simulink model "stm32f0_ccp_sensor"  (Simulink 7.3)
settings: Solver=ode3  SolverMode=SingleTasking  StartTime=0.0  StopTime=10.0  RelTol=1e-3
PreLoadFcn:
  | waijung.modelPreload; % Required for working with Waijung Blockset. Do not remove.
undefined symbols (not defined in the file): ARM, LQFP48, MDK, STM32F072CB
libraries: simulink x216, waijung_soft_i2c_lib x28, waijung_addon_module x12, stm32f0_flash_lib x10, stm32f0_can_lib x3, stm32f0_reset_lib x1, waijung_crc_lib x1, stm32f0_boot_lib x1, stm32f0_device_config_lib x1
(part 2 of 6)

== system stm32f0_ccp_sensor/CCP Handler/CRO CONNECT Parser ==
  Data(8) : Inport  OutDataType=fixdt(1, 16)  OutScaling=2^0
  CONNECT Handler : Subsystem  TreatAsAtomicUnit=on
  Demux : Demux  Outputs=8
  Mux : Mux  Inputs=6
  Terminator : Terminator
  Connected : Outport  OutDataType=fixdt(1, 16)  OutScaling=2^0
  CMD : Outport  Port=2  OutDataType=fixdt(1, 16)  OutScaling=2^0
  Data(6) : Outport  Port=3  OutDataType=fixdt(1, 16)  OutScaling=2^0
  CTR : Outport  Port=4  OutDataType=fixdt(1, 16)  OutScaling=2^0
  wires:
  Data(8)/1 -> Demux/1
  Demux/1 -> CMD/1, CONNECT Handler/1(CMD)
  Demux/3 -> CONNECT Handler/2(Station Addr LSB), Mux/1
  Demux/4 -> CONNECT Handler/3(Station Addr MSB), Mux/2
  CONNECT Handler/1(Connected) -> Connected/1
  CONNECT Handler/2(Station Address) -> Terminator/1
  Demux/8 -> Mux/6
  Demux/7 -> Mux/5
  Demux/6 -> Mux/4
  Demux/5 -> Mux/3
  Mux/1 -> Data(6)/1
  Demux/2 -> CTR/1

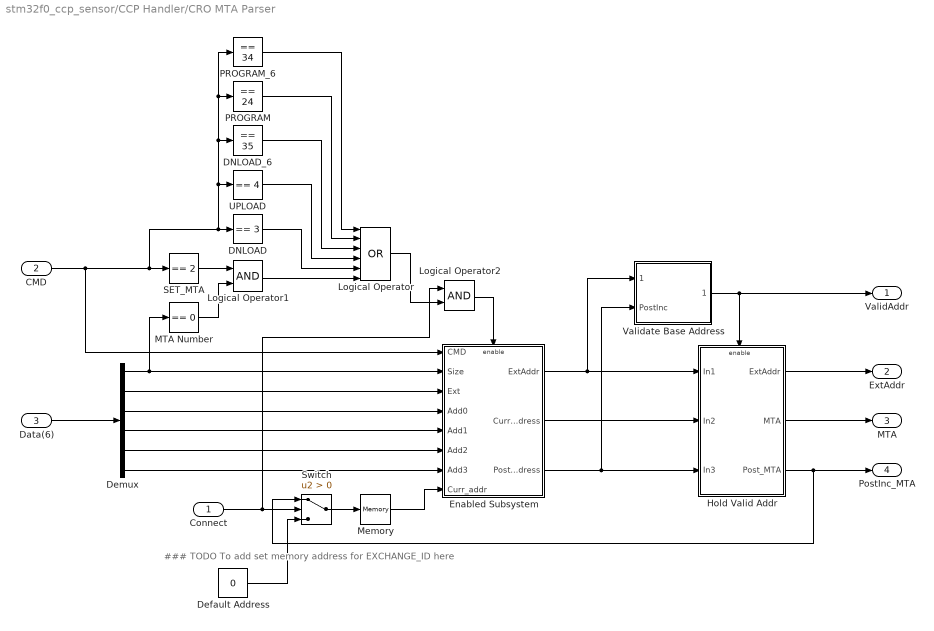
== system stm32f0_ccp_sensor/CCP Handler/CRO MTA Parser ==
  note: ### TODO
      | To add set memory address for EXCHANGE_ID here
  Connect : Inport  OutDataType=fixdt(1, 16)  OutScaling=2^0
  CMD : Inport  Port=2  OutDataType=fixdt(1, 16)  OutScaling=2^0
  Data(6) : Inport  Port=3  OutDataType=fixdt(1, 16)  OutScaling=2^0
  DNLOAD : simulink/Logic and Bit Operations/Compare To Constant  SystemSampleTime=-1  relop===  const=3  LogicOutDataTypeMode=uint8  ZeroCross=off
  DNLOAD_6 : simulink/Logic and Bit Operations/Compare To Constant  SystemSampleTime=-1  relop===  const=35  LogicOutDataTypeMode=uint8  ZeroCross=off
  Default Address : Constant  Value=0  OutDataTypeMode=uint32  OutDataType=fixdt(1, 16)  OutScaling=2^0  OutDataTypeStr=uint32
  Demux : Demux  Outputs=6
  Enabled Subsystem : Subsystem  TreatAsAtomicUnit=on
  Hold Valid Addr : Subsystem
  Logical Operator : Logic  Operator=OR  Inputs=6  AllPortsSameDT=off  OutDataTypeMode=boolean  LogicDataType=fixdt(0, 8)  OutDataTypeStr=boolean
  Logical Operator1 : Logic  AllPortsSameDT=off  OutDataTypeMode=boolean  LogicDataType=fixdt(0, 8)  OutDataTypeStr=boolean
  Logical Operator2 : Logic  AllPortsSameDT=off  OutDataTypeMode=boolean  LogicDataType=fixdt(0, 8)  OutDataTypeStr=boolean
  MTA Number : simulink/Logic and Bit Operations/Compare To Constant  SystemSampleTime=-1  relop===  const=0  LogicOutDataTypeMode=uint8  ZeroCross=off
  Memory : Memory  InheritSampleTime=on  LinearizeMemory=on
  PROGRAM : simulink/Logic and Bit Operations/Compare To Constant  SystemSampleTime=-1  relop===  const=24  LogicOutDataTypeMode=uint8  ZeroCross=off
  PROGRAM_6 : simulink/Logic and Bit Operations/Compare To Constant  SystemSampleTime=-1  relop===  const=34  LogicOutDataTypeMode=uint8  ZeroCross=off
  SET_MTA : simulink/Logic and Bit Operations/Compare To Constant  SystemSampleTime=-1  relop===  const=2  LogicOutDataTypeMode=uint8  ZeroCross=off
  Switch : Switch  Criteria=u2 > Threshold  OutDataType=fixdt(1, 16)  OutScaling=2^0
  UPLOAD : simulink/Logic and Bit Operations/Compare To Constant  SystemSampleTime=-1  relop===  const=4  LogicOutDataTypeMode=uint8  ZeroCross=off
  Validate Base Address : Subsystem
  ValidAddr : Outport  OutDataType=fixdt(1, 16)  OutScaling=2^0
  ExtAddr : Outport  Port=2  OutDataType=fixdt(1, 16)  OutScaling=2^0
  MTA : Outport  Port=3  OutDataType=fixdt(1, 16)  OutScaling=2^0
  PostInc_MTA : Outport  Port=4  OutDataType=fixdt(1, 16)  OutScaling=2^0
  wires:
  Data(6)/1 -> Demux/1
  CMD/1 -> SET_MTA/1, DNLOAD/1, UPLOAD/1, DNLOAD_6/1, PROGRAM/1, PROGRAM_6/1, Enabled Subsystem/1(CMD)
  Demux/1 -> MTA Number/1, Enabled Subsystem/2(Size)
  MTA Number/1 -> Logical Operator1/2
  SET_MTA/1 -> Logical Operator1/1
  Demux/3 -> Enabled Subsystem/4(Add0)
  Demux/4 -> Enabled Subsystem/5(Add1)
  Demux/5 -> Enabled Subsystem/6(Add2)
  Demux/6 -> Enabled Subsystem/7(Add3)
  Demux/2 -> Enabled Subsystem/3(Ext)
  Enabled Subsystem/2(Curr_Address) -> Hold Valid Addr/2(In2)
  Logical Operator1/1 -> Logical Operator/6
  PROGRAM_6/1 -> Logical Operator/1
  PROGRAM/1 -> Logical Operator/2
  DNLOAD_6/1 -> Logical Operator/3
  UPLOAD/1 -> Logical Operator/4
  DNLOAD/1 -> Logical Operator/5
  Enabled Subsystem/3(Post_Address) -> Hold Valid Addr/3(In3), Validate Base Address/2(PostInc)
  Memory/1 -> Enabled Subsystem/8(Curr_addr)
  Switch/1 -> Memory/1
  Connect/1 -> Switch/2, Logical Operator2/1
  Default Address/1 -> Switch/3
  Logical Operator2/1 -> Enabled Subsystem/Enable
  Logical Operator/1 -> Logical Operator2/2
  Enabled Subsystem/1(ExtAddr) -> Hold Valid Addr/1(In1), Validate Base Address/1(ExtAddr)
  Hold Valid Addr/1(ExtAddr) -> ExtAddr/1
  Hold Valid Addr/2(MTA) -> MTA/1
  Hold Valid Addr/3(Post_MTA) -> PostInc_MTA/1, Switch/1
  Validate Base Address/1(ValidAddr) -> Hold Valid Addr/Enable, ValidAddr/1

== system stm32f0_ccp_sensor/CCP Handler/CRO UNLOCK Parser ==
  Connect : Inport  OutDataType=fixdt(1, 16)  OutScaling=2^0
  CMD : Inport  Port=2  OutDataType=fixdt(1, 16)  OutScaling=2^0
  Data(6) : Inport  Port=3  OutDataType=fixdt(1, 16)  OutScaling=2^0
  Constant : Constant  Value=[0 0 0]  OutDataTypeMode=uint8  OutDataType=fixdt(1, 16)  OutScaling=2^0  OutDataTypeStr=uint8
  Demux : Demux  Outputs=3
  Enabled Subsystem : Subsystem  TreatAsAtomicUnit=on
  Memory : Memory
  Switch : Switch  Criteria=u2 > Threshold  OutDataType=fixdt(1, 16)  OutScaling=2^0
  CAL Unlocked : Outport  OutDataType=fixdt(1, 16)  OutScaling=2^0
  PGM Unlocked : Outport  Port=2  OutDataType=fixdt(1, 16)  OutScaling=2^0
  DAQ Unlocked : Outport  Port=3  OutDataType=fixdt(1, 16)  OutScaling=2^0
  wires:
  Connect/1 -> Switch/2, Enabled Subsystem/Enable
  Constant/1 -> Switch/3
  Switch/1 -> Demux/1, Memory/1
  Demux/1 -> CAL Unlocked/1
  Demux/2 -> PGM Unlocked/1
  Demux/3 -> DAQ Unlocked/1
  Memory/1 -> Enabled Subsystem/3(Last status)
  Data(6)/1 -> Enabled Subsystem/2(Data(6))
  CMD/1 -> Enabled Subsystem/1(CMD)
  Enabled Subsystem/1(Out1) -> Switch/1

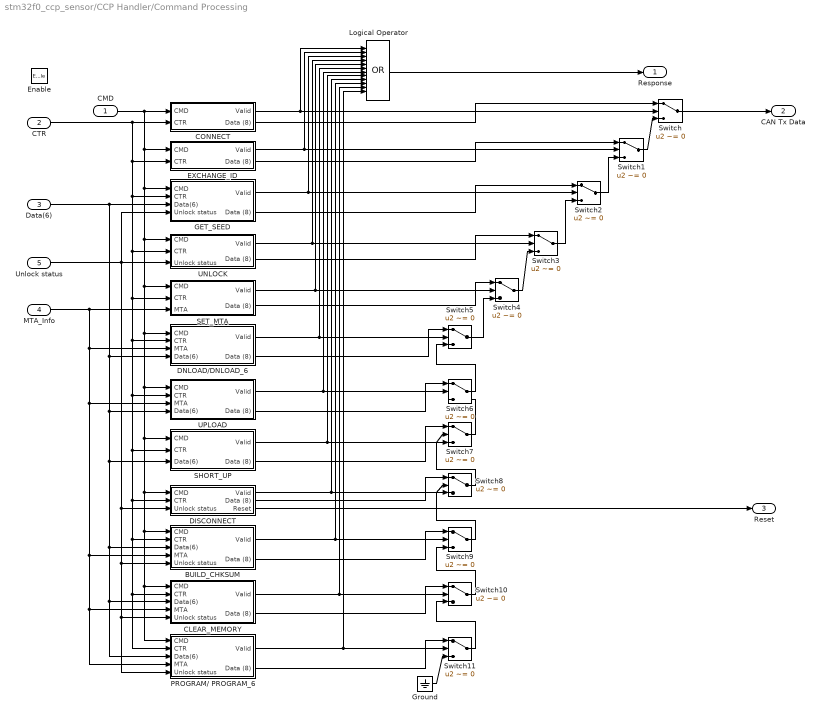
== system stm32f0_ccp_sensor/CCP Handler/Command Processing ==
  CMD : Inport  OutDataType=fixdt(1, 16)  OutScaling=2^0
  CTR : Inport  Port=2  OutDataType=fixdt(1, 16)  OutScaling=2^0
  Data(6) : Inport  Port=3  OutDataType=fixdt(1, 16)  OutScaling=2^0
  MTA_Info : Inport  Port=4  OutDataType=fixdt(1, 16)  OutScaling=2^0
  Unlock status : Inport  Port=5  OutDataType=fixdt(1, 16)  OutScaling=2^0
  Enable : EnablePort
  BUILD_CHKSUM : Subsystem
  CLEAR_MEMORY : Subsystem
  CONNECT : Subsystem
  DISCONNECT : Subsystem
  DNLOAD/DNLOAD_6 : Subsystem
  EXCHANGE_ID : Subsystem
  GET_SEED : Subsystem
  Ground : Ground
  Logical Operator : Logic  Operator=OR  Inputs=12  AllPortsSameDT=off  OutDataTypeMode=boolean  LogicDataType=fixdt(0, 8)  OutDataTypeStr=boolean
  PROGRAM/ PROGRAM_6 : Subsystem
  SET_MTA : Subsystem
  SHORT_UP : Subsystem
  Switch{,1..11} (12 alike) : Switch  Criteria=u2 ~= 0  OutDataType=fixdt(1, 16)  OutScaling=2^0
  UNLOCK : Subsystem
  UPLOAD : Subsystem
  Response : Outport  OutDataType=fixdt(1, 16)  OutScaling=2^0
  CAN Tx Data : Outport  Port=2  OutDataType=fixdt(1, 16)  OutScaling=2^0  InitialOutput=[0 0 0 0 0 0 0 0]
  Reset : Outport  Port=3  OutDataType=fixdt(1, 16)  OutScaling=2^0  InitialOutput=0
  wires:
  CMD/1 -> CONNECT/1(CMD), EXCHANGE_ID/1(CMD), GET_SEED/1(CMD), UNLOCK/1(CMD), SET_MTA/1(CMD), UPLOAD/1(CMD), SHORT_UP/1(CMD), DISCONNECT/1(CMD), BUILD_CHKSUM/1(CMD), CLEAR_MEMORY/1(CMD), PROGRAM/ PROGRAM_6/1(CMD), DNLOAD/DNLOAD_6/1(CMD)
  Switch/1 -> CAN Tx Data/1
  CTR/1 -> CONNECT/2(CTR), EXCHANGE_ID/2(CTR), GET_SEED/2(CTR), UNLOCK/2(CTR), SET_MTA/2(CTR), DNLOAD/DNLOAD_6/2(CTR), UPLOAD/2(CTR), SHORT_UP/2(CTR), DISCONNECT/2(CTR), BUILD_CHKSUM/2(CTR), CLEAR_MEMORY/2(CTR), PROGRAM/ PROGRAM_6/2(CTR)
  CONNECT/1(Valid) -> Logical Operator/1, Switch/2
  EXCHANGE_ID/1(Valid) -> Logical Operator/2, Switch1/2
  Data(6)/1 -> GET_SEED/3(Data(6)), DNLOAD/DNLOAD_6/4(Data(6)), UPLOAD/4(Data(6)), SHORT_UP/3(Data(6)), BUILD_CHKSUM/3(Data(6)), CLEAR_MEMORY/3(Data(6)), PROGRAM/ PROGRAM_6/3(Data(6))
  GET_SEED/1(Valid) -> Logical Operator/3, Switch2/2
  Switch2/1 -> Switch1/3
  GET_SEED/2(Data (8)) -> Switch2/1
  EXCHANGE_ID/2(Data (8)) -> Switch1/1
  CONNECT/2(Data (8)) -> Switch/1
  Switch1/1 -> Switch/3
  Logical Operator/1 -> Response/1
  Unlock status/1 -> GET_SEED/4(Unlock status), UNLOCK/3(Unlock status), BUILD_CHKSUM/5(Unlock status), CLEAR_MEMORY/5(Unlock status), PROGRAM/ PROGRAM_6/5(Unlock status), DISCONNECT/3(Unlock status)
  UNLOCK/1(Valid) -> Logical Operator/4, Switch3/2
  Switch3/1 -> Switch2/3
  UNLOCK/2(Data (8)) -> Switch3/1
  SET_MTA/1(Valid) -> Logical Operator/5, Switch4/2
  Switch4/1 -> Switch3/3
  SET_MTA/2(Data (8)) -> Switch4/1
  MTA_Info/1 -> SET_MTA/3(MTA), DNLOAD/DNLOAD_6/3(MTA), UPLOAD/3(MTA), BUILD_CHKSUM/4(MTA), CLEAR_MEMORY/4(MTA), PROGRAM/ PROGRAM_6/4(MTA)
  DNLOAD/DNLOAD_6/1(Valid) -> Logical Operator/6, Switch5/2
  Switch5/1 -> Switch4/3
  DNLOAD/DNLOAD_6/2(Data (8)) -> Switch5/1
  UPLOAD/1(Valid) -> Logical Operator/7, Switch6/2
  Switch6/1 -> Switch5/3
  UPLOAD/2(Data (8)) -> Switch6/1
  SHORT_UP/1(Valid) -> Logical Operator/8, Switch7/2
  Switch7/1 -> Switch6/3
  SHORT_UP/2(Data (8)) -> Switch7/1
  DISCONNECT/1(Valid) -> Logical Operator/9, Switch8/2
  Switch8/1 -> Switch7/3
  DISCONNECT/2(Data (8)) -> Switch8/1
  BUILD_CHKSUM/1(Valid) -> Logical Operator/10, Switch9/2
  BUILD_CHKSUM/2(Data (8)) -> Switch9/1
  Switch9/1 -> Switch8/3
  CLEAR_MEMORY/1(Valid) -> Logical Operator/11, Switch10/2
  Switch10/1 -> Switch9/3
  CLEAR_MEMORY/2(Data (8)) -> Switch10/1
  PROGRAM/ PROGRAM_6/1(Valid) -> Logical Operator/12, Switch11/2
  PROGRAM/ PROGRAM_6/2(Data (8)) -> Switch11/1
  Switch11/1 -> Switch10/3
  Ground/1 -> Switch11/3
  DISCONNECT/3(Reset) -> Reset/1

== system stm32f0_ccp_sensor/HIH6131/Read ==
  In1 : Inport
  Enable : EnablePort
  Compare To Zero : simulink/Logic and Bit Operations/Compare To Zero  SystemSampleTime=-1  relop===  LogicOutDataTypeMode=boolean  ZeroCross=off
  Constant1 : Constant  Value=40  OutDataTypeMode=single  OutDataType=fixdt(1, 16)  OutScaling=2^0  OutDataTypeStr=single
  Data Type Conversion3 : DataTypeConversion  OutDataTypeMode=single  OutDataType=fixdt(1, 16)  OutScaling=2^0  OutDataTypeStr=single
  Data Type Conversion4 : DataTypeConversion  OutDataTypeMode=single  OutDataType=fixdt(1, 16)  OutScaling=2^0  OutDataTypeStr=single
  Gain : Gain  Gain=100/16382  ParameterDataType=fixdt(1, 16)  ParameterScaling=2^0  OutDataType=fixdt(1, 16)  OutScaling=2^0
  Gain1 : Gain  Gain=165/16382  ParameterDataType=fixdt(1, 16)  ParameterScaling=2^0  OutDataType=fixdt(1, 16)  OutScaling=2^0
  Mux : Mux
  Soft I2C Master Read/Write : waijung_soft_i2c_lib/Soft I2C Master Read//Write  conf=ReadWrite  targetname=stm32f0  module=1  transfer=Blocking  clk=100  timeout=25  sdapins={'A4','A6'}  sclpins='A5'  writecount=0  readcount=4  waittime=0  forcestop=off  portpinstr=0  sampletime=inf  blockid=HIH6131ReadSoftI2CMasterReadWrite  inputporttype=[3]  inputportwidth=[]  inputportlabel={'SlvAddr'}  outputporttype="[3 3 3 3 3    ]"  outputportwidth=[1 1 1 1 1]  outputportlabel={'Status' 'Rd0 (uint8)' 'Rd1 (uint8)' 'Rd2 (uint8)' 'Rd3 (uint8)'}  compat=0  optionstring="[\"1\",\"0\",\"4\",\"0\",\"off\",\"1\"]"
  Subsystem : Subsystem
  Subtract : Sum  Inputs=+-  OutDataType=fixdt(1, 16)  OutScaling=2^-10
  Terminator : Terminator
  Humid : Outport  OutDataType=fixdt(1, 16)  OutScaling=2^0
  Temp : Outport  Port=2  OutDataType=fixdt(1, 16)  OutScaling=2^0
  wires:
  Soft I2C Master Read/Write/2 -> Mux/1
  Soft I2C Master Read/Write/3 -> Mux/2
  Soft I2C Master Read/Write/4 -> Mux/3
  Soft I2C Master Read/Write/5 -> Mux/4
  Mux/1 -> Subsystem/1(In1)
  Compare To Zero/1 -> Subsystem/Enable
  Soft I2C Master Read/Write/1 -> Compare To Zero/1
  Subsystem/2(Humidity) -> Data Type Conversion3/1
  Subsystem/3(Temperature) -> Data Type Conversion4/1
  Gain1/1 -> Subtract/1
  Constant1/1 -> Subtract/2
  Subsystem/1(Status) -> Terminator/1
  Subtract/1 -> Temp/1
  Data Type Conversion3/1 -> Gain/1
  Data Type Conversion4/1 -> Gain1/1
  Gain/1 -> Humid/1
  In1/1 -> Soft I2C Master Read/Write/1

== system stm32f0_ccp_sensor/HIH6131/Request ==
  In1 : Inport
  Enable : EnablePort
  Soft I2C Master Read/Write : waijung_soft_i2c_lib/Soft I2C Master Read//Write  conf=ReadWrite  targetname=stm32f0  module=1  transfer=Blocking  clk=100  timeout=25  sdapins={'A4','A6'}  sclpins='A5'  writecount=0  readcount=0  waittime=0  forcestop=off  portpinstr=0  sampletime=inf  blockid=HIH6131RequestSoftI2CMasterReadWrite  inputporttype=[3]  inputportwidth=[]  inputportlabel={'SlvAddr'}  outputporttype=[3]  outputportwidth=[1]  outputportlabel={'Status'}  compat=0  optionstring="[\"1\",\"0\",\"0\",\"0\",\"off\",\"1\"]"
  Terminator : Terminator
  wires:
  In1/1 -> Soft I2C Master Read/Write/1
  Soft I2C Master Read/Write/1 -> Terminator/1

== system stm32f0_ccp_sensor/MAX44009/Enabled Subsystem ==
  note: # E
  note: #M
  Configuration : Inport  OutDataType=fixdt(1, 16)  OutScaling=2^0
  MSB : Inport  Port=2  OutDataType=fixdt(1, 16)  OutScaling=2^0
  LSB : Inport  Port=3  OutDataType=fixdt(1, 16)  OutScaling=2^0
  Enable : EnablePort
  Bitwise Operator : simulink/Logic and Bit Operations/Bitwise Operator  logicop=OR  UseBitMask=off  NumInputPorts=2  BitMask=bin2dec('11011001')  BitMaskRealWorld=Stored Integer
  Bitwise Operator1 : simulink/Logic and Bit Operations/Bitwise Operator  logicop=AND  UseBitMask=on  BitMask=hex2dec('F')  BitMaskRealWorld=Stored Integer
  CDR_ : simulink/Logic and Bit Operations/Bitwise Operator  logicop=AND  UseBitMask=on  BitMask=8  BitMaskRealWorld=Stored Integer
  Compare To Zero : simulink/Logic and Bit Operations/Compare To Zero  SystemSampleTime=-1  relop=~=  LogicOutDataTypeMode=uint8  ZeroCross=off
  Constant1 : Constant  Value=0.045  OutDataType=fixdt(1, 16)  OutScaling=2^0
  Constant2 : Constant  Value=2  OutDataTypeMode=single  OutDataType=fixdt(1, 16)  OutScaling=2^0  OutDataTypeStr=single
  Data Type Conversion{,1..3} (4 alike) : DataTypeConversion  OutDataTypeMode=single  OutDataType=fixdt(1, 16)  OutScaling=2^0  OutDataTypeStr=single
  Math Function : Math  Operator=pow  OutDataType=fixdt(1, 16)  OutScaling=2^0  SaturateOnIntegerOverflow=on
  Product : Product  Inputs=3  OutDataType=fixdt(1, 16)  OutScaling=2^0  RndMeth=Zero  OutDataTypeStr=Inherit: Same as first input
  Shift Arithmetic : simulink/Logic and Bit Operations/Shift Arithmetic  SystemSampleTime=-1  nBitShiftRight=4  nBinPtShiftRight=0
  Shift Arithmetic1 : simulink/Logic and Bit Operations/Shift Arithmetic  SystemSampleTime=-1  nBitShiftRight=-4  nBinPtShiftRight=0
  Lux : Outport  OutDataType=fixdt(1, 16)  OutScaling=2^0
  CDR : Outport  Port=2  OutDataType=fixdt(1, 16)  OutScaling=2^0
  wires:
  Compare To Zero/1 -> CDR/1
  CDR_/1 -> Compare To Zero/1
  Data Type Conversion2/1 -> Product/1
  Data Type Conversion/1 -> Product/2
  Bitwise Operator1/1 -> Data Type Conversion3/1
  Constant1/1 -> Data Type Conversion2/1
  Math Function/1 -> Data Type Conversion/1
  MSB/1 -> Shift Arithmetic/1, Shift Arithmetic1/1
  Shift Arithmetic/1 -> Bitwise Operator1/1
  Shift Arithmetic1/1 -> Bitwise Operator/1
  LSB/1 -> Bitwise Operator/2
  Bitwise Operator/1 -> Data Type Conversion1/1
  Data Type Conversion1/1 -> Product/3
  Configuration/1 -> CDR_/1
  Product/1 -> Lux/1
  Constant2/1 -> Math Function/1
  Data Type Conversion3/1 -> Math Function/2

== system stm32f0_ccp_sensor/MPL3115A2/Convert ==
  In1 : Inport
  In2 : Inport  Port=2
  In3 : Inport  Port=3
  Enable : EnablePort
  Add : Sum  OutDataType=fixdt(1, 16)  OutScaling=2^-10
  Bitwise Operator : simulink/Logic and Bit Operations/Bitwise Operator  logicop=OR  UseBitMask=off  NumInputPorts=3  BitMask=bin2dec('11011001')  BitMaskRealWorld=Stored Integer
  Bitwise Operator1 : simulink/Logic and Bit Operations/Bitwise Operator  logicop=AND  UseBitMask=on  BitMask=3  BitMaskRealWorld=Stored Integer
  Data Type Conversion{,1..2,4} (4 alike) : DataTypeConversion  OutDataTypeMode=uint32  OutDataType=fixdt(1, 16)  OutScaling=2^0  OutDataTypeStr=uint32
  Data Type Conversion3 : DataTypeConversion  OutDataTypeMode=single  OutDataType=fixdt(1, 16)  OutScaling=2^0  OutDataTypeStr=single
  Data Type Conversion6 : DataTypeConversion  OutDataTypeMode=single  OutDataType=fixdt(1, 16)  OutScaling=2^0  OutDataTypeStr=single
  Gain : Gain  Gain=0.25  ParameterDataType=fixdt(1, 16)  ParameterScaling=2^0  OutDataTypeMode=single  OutDataType=fixdt(1, 16)  OutScaling=2^0  OutDataTypeStr=single
  Shift Arithmetic : simulink/Logic and Bit Operations/Shift Arithmetic  SystemSampleTime=-1  nBitShiftRight=-10  nBinPtShiftRight=0
  Shift Arithmetic1 : simulink/Logic and Bit Operations/Shift Arithmetic  SystemSampleTime=-1  nBitShiftRight=4  nBinPtShiftRight=0
  Shift Arithmetic2 : simulink/Logic and Bit Operations/Shift Arithmetic  SystemSampleTime=-1  nBitShiftRight=-2  nBinPtShiftRight=0
  Shift Arithmetic3 : simulink/Logic and Bit Operations/Shift Arithmetic  SystemSampleTime=-1  nBitShiftRight=6  nBinPtShiftRight=0
  Pa : Outport  OutDataType=fixdt(1, 16)  OutScaling=2^0
  wires:
  Shift Arithmetic3/1 -> Bitwise Operator/3
  Data Type Conversion4/1 -> Shift Arithmetic3/1
  Shift Arithmetic2/1 -> Bitwise Operator/2
  In3/1 -> Data Type Conversion4/1, Shift Arithmetic1/1
  In2/1 -> Data Type Conversion1/1
  Add/1 -> Pa/1
  In1/1 -> Data Type Conversion/1
  Data Type Conversion6/1 -> Add/2
  Gain/1 -> Data Type Conversion6/1
  Data Type Conversion3/1 -> Add/1
  Bitwise Operator1/1 -> Gain/1
  Shift Arithmetic1/1 -> Bitwise Operator1/1
  Data Type Conversion2/1 -> Data Type Conversion3/1
  Bitwise Operator/1 -> Data Type Conversion2/1
  Data Type Conversion1/1 -> Shift Arithmetic2/1
  Shift Arithmetic/1 -> Bitwise Operator/1
  Data Type Conversion/1 -> Shift Arithmetic/1

== system stm32f0_ccp_sensor/MPL3115A2/MPL3115A2_Initialize ==
  SlvAddr : Inport  OutDataType=fixdt(1, 16)  OutScaling=2^0
  CNTRL_REG1 : Constant  Value=hex2dec('26')  OutDataTypeMode=uint8  OutDataType=fixdt(1, 16)  OutScaling=2^0  OutDataTypeStr=uint8
  Compare To Constant : simulink/Logic and Bit Operations/Compare To Constant  SystemSampleTime=-1  relop===  const=7  LogicOutDataTypeMode=boolean  ZeroCross=off
  Compare To Constant1 : simulink/Logic and Bit Operations/Compare To Constant  SystemSampleTime=-1  relop===  const=hex2dec('39')  LogicOutDataTypeMode=boolean  ZeroCross=off
  Compare To Zero : simulink/Logic and Bit Operations/Compare To Zero  SystemSampleTime=-1  relop===  LogicOutDataTypeMode=boolean  ZeroCross=off
  Compare To Zero1 : simulink/Logic and Bit Operations/Compare To Zero  SystemSampleTime=-1  relop===  LogicOutDataTypeMode=boolean  ZeroCross=off
  Logical Operator1 : Logic  Inputs=4  AllPortsSameDT=off  OutDataTypeMode=boolean  LogicDataType=fixdt(0, 8)  OutDataTypeStr=boolean
  Logical Operator2 : Logic  Inputs=3  AllPortsSameDT=off  OutDataTypeMode=boolean  LogicDataType=fixdt(0, 8)  OutDataTypeStr=boolean
  Logical Operator3 : Logic  Operator=NOT  Inputs=4  AllPortsSameDT=off  OutDataTypeMode=boolean  LogicDataType=fixdt(0, 8)  OutDataTypeStr=boolean
  Logical Operator4 : Logic  Operator=NOT  Inputs=4  AllPortsSameDT=off  OutDataTypeMode=boolean  LogicDataType=fixdt(0, 8)  OutDataTypeStr=boolean
  Logical Operator5 : Logic  Operator=OR  AllPortsSameDT=off  OutDataTypeMode=boolean  LogicDataType=fixdt(0, 8)  OutDataTypeStr=boolean
  PT_DATA_CFG : Constant  Value=hex2dec('13')  OutDataTypeMode=uint8  OutDataType=fixdt(1, 16)  OutScaling=2^0  OutDataTypeStr=uint8
  Soft I2C Master Read/Write : waijung_soft_i2c_lib/Soft I2C Master Read//Write  conf=ReadWrite  targetname=stm32f0  module=1  transfer=Blocking  clk=100  timeout=25  sdapins={'A4','A6'}  sclpins='A5'  writecount=1  readcount=1  waittime=0  forcestop=off  portpinstr=0  sampletime=inf  blockid=MPL3115A2MPL3115A2_InitializeSoftI2CMasterReadWrite  inputporttype=[3 3]  inputportwidth=[]  inputportlabel={'SlvAddr' 'Wr0 (uint8)'}  outputporttype=[3 3 ]  outputportwidth=[1 1]  outputportlabel={'Status' 'Rd0 (uint8)'}  compat=0  optionstring="[\"1\",\"1\",\"1\",\"0\",\"off\",\"1\"]"
  Soft I2C Master Read/Write1 : waijung_soft_i2c_lib/Soft I2C Master Read//Write  conf=ReadWrite  targetname=stm32f0  module=1  transfer=Blocking  clk=100  timeout=25  sdapins={'A4','A6'}  sclpins='A5'  writecount=1  readcount=1  waittime=0  forcestop=off  portpinstr=0  sampletime=inf  blockid=MPL3115A2MPL3115A2_InitializeSoftI2CMasterReadWrite1  inputporttype=[3 3]  inputportwidth=[]  inputportlabel={'SlvAddr' 'Wr0 (uint8)'}  outputporttype=[3 3 ]  outputportwidth=[1 1]  outputportlabel={'Status' 'Rd0 (uint8)'}  compat=0  optionstring="[\"1\",\"1\",\"1\",\"0\",\"off\",\"1\"]"
  Write Configure : Subsystem  TreatAsAtomicUnit=on
  SETUP_READY : Outport  OutDataType=fixdt(1, 16)  OutScaling=2^0
  wires:
  Logical Operator1/1 -> SETUP_READY/1
  Logical Operator5/1 -> Logical Operator2/3
  Logical Operator3/1 -> Logical Operator5/1
  Logical Operator4/1 -> Logical Operator5/2
  Logical Operator2/1 -> Write Configure/Enable
  Compare To Constant/1 -> Logical Operator4/1, Logical Operator1/4
  Compare To Zero1/1 -> Logical Operator2/2, Logical Operator1/3
  Compare To Constant1/1 -> Logical Operator3/1, Logical Operator1/2
  Soft I2C Master Read/Write/2 -> Compare To Constant1/1
  Soft I2C Master Read/Write1/2 -> Compare To Constant/1
  Compare To Zero/1 -> Logical Operator2/1, Logical Operator1/1
  Soft I2C Master Read/Write1/1 -> Compare To Zero1/1
  Soft I2C Master Read/Write/1 -> Compare To Zero/1
  PT_DATA_CFG/1 -> Soft I2C Master Read/Write1/2
  CNTRL_REG1/1 -> Soft I2C Master Read/Write/2
  SlvAddr/1 -> Write Configure/1(SlvAddr), Soft I2C Master Read/Write1/1, Soft I2C Master Read/Write/1

== system stm32f0_ccp_sensor/MPL3115A2/Reading ==
  SlvAddr : Inport  OutDataType=fixdt(1, 16)  OutScaling=2^0
  Enable : EnablePort
  Bitwise Operator : simulink/Logic and Bit Operations/Bitwise Operator  logicop=AND  UseBitMask=on  BitMask=8  BitMaskRealWorld=Stored Integer
  Compare To Zero : simulink/Logic and Bit Operations/Compare To Zero  SystemSampleTime=-1  relop===  LogicOutDataTypeMode=boolean  ZeroCross=off
  Compare To Zero2 : simulink/Logic and Bit Operations/Compare To Zero  SystemSampleTime=-1  relop=~=  LogicOutDataTypeMode=boolean  ZeroCross=off
  Logical Operator : Logic  AllPortsSameDT=off  OutDataTypeMode=boolean  LogicDataType=fixdt(0, 8)  OutDataTypeStr=boolean
  STATUS : Constant  Value=0  OutDataTypeMode=uint8  OutDataType=fixdt(1, 16)  OutScaling=2^0  OutDataTypeStr=uint8
  Soft I2C Master Read/Write : waijung_soft_i2c_lib/Soft I2C Master Read//Write  conf=ReadWrite  targetname=stm32f0  module=1  transfer=Blocking  clk=100  timeout=25  sdapins={'A4','A6'}  sclpins='A5'  writecount=1  readcount=6  waittime=0  forcestop=off  portpinstr=0  sampletime=inf  blockid=MPL3115A2ReadingSoftI2CMasterReadWrite  inputporttype=[3 3]  inputportwidth=[]  inputportlabel={'SlvAddr' 'Wr0 (uint8)'}  outputporttype="[3 3 3 3 3 3 3      ]"  outputportwidth=[1 1 1 1 1 1 1]  outputportlabel={'Status' 'Rd0 (uint8)' 'Rd1 (uint8)' 'Rd2 (uint8)' 'Rd3 (uint8)' 'Rd4 (uint8)' 'Rd5 (uint8)'}  compat=0  optionstring="[\"1\",\"1\",\"6\",\"0\",\"off\",\"1\"]"
  DATA_VALID : Outport  OutDataType=fixdt(1, 16)  OutScaling=2^0
  P_MSB : Outport  Port=2  OutDataType=fixdt(1, 16)  OutScaling=2^0
  P_CSB : Outport  Port=3  OutDataType=fixdt(1, 16)  OutScaling=2^0
  P_LSB : Outport  Port=4  OutDataType=fixdt(1, 16)  OutScaling=2^0
  T_MSB : Outport  Port=5  OutDataType=fixdt(1, 16)  OutScaling=2^0
  T_LSB : Outport  Port=6  OutDataType=fixdt(1, 16)  OutScaling=2^0
  wires:
  Soft I2C Master Read/Write/7 -> T_LSB/1
  Soft I2C Master Read/Write/6 -> T_MSB/1
  Soft I2C Master Read/Write/5 -> P_LSB/1
  Soft I2C Master Read/Write/4 -> P_CSB/1
  Soft I2C Master Read/Write/3 -> P_MSB/1
  Compare To Zero/1 -> Logical Operator/1
  Soft I2C Master Read/Write/2 -> Bitwise Operator/1
  Soft I2C Master Read/Write/1 -> Compare To Zero/1
  Logical Operator/1 -> DATA_VALID/1
  Compare To Zero2/1 -> Logical Operator/2
  Bitwise Operator/1 -> Compare To Zero2/1
  STATUS/1 -> Soft I2C Master Read/Write/2
  SlvAddr/1 -> Soft I2C Master Read/Write/1

== system stm32f0_ccp_sensor/Network/Interface Configuration/CAN_ID Configuration ==
  note: ### Set ID via UART
      | Format: 'canid_set=%u\r\n'
  Enabled Subsystem : Subsystem  TreatAsAtomicUnit=on
  UART Rx : S-Function  FunctionName=stm32f0_uart  Parameters=conf,inputporttype,inputportwidth,outputporttype,outputportwidth,asciiheader,optionstring,headerstring,terminatorstring,asciidatatypestring,sampletime,blockid  EnableBusSupport=off  mask(stm32f0_uart){conf=Rx, uartmodule=1, baudrate=115200, databits=8, parity=No, stopbit=1, remaptxpin=A9, remaprxpin=A10, flowcontrol=None, remapctspin=Not used, remaprtspin=Not used, advanceoptions=off, rxbuffersize=64, txbuffersize=64, transfer=Non-Blocking, packetmode=Ascii, binheader='7E 7E', binterminator='03 03', porttype_double=0, porttype_single=0, porttype_int8=0, porttype_uint8=0, porttype_int16=0, porttype_uint16=0, porttype_int32=0, porttype_uint32=2, asciiformat='canid_set=%u', rx_asciiterminator=CRLF (0x0D 0x0A - "\r\n"), tx_asciiterminator=LF (0x0A - "\n"), storagename=<empty>, varname=, asciiheader=canid_set=%u\r\n, sampletime=inf, enablecustomportlabel=off, cinputportlabel=de, coutputportlabel=fff,ff,sdfsd, portpinstr=0, blockid=NetworkInterfaceConfigurationCAN_IDConfigurationUARTRx, inputporttype=[], inputportwidth=[], inputportlabel={}, outputporttype=[3  7], outputportwidth=[], outputportlabel={'READY'  '%u'}, compat=0, optionstring=["1", "1", "A", "9", "1", "A", "10", "0", "*", "*", "0", "*", "*", "1", "1", "", "", "115200", "8", "No", "1", "None", "3", "2", "64", "64", "Ascii", "Non-Blocking", ""], headerstring=[], terminatorstring=["13","10"], asciidatatypestring=["uint32_t"], lastmodule=1}
      mask prompts: conf "Configuration"; uartmodule "UART Module"; baudrate "Baud rate (bps)"; databits "Data bits"; stopbit "Stop bit"; remaptxpin "Tx pin"; remaprxpin "Rx pin"; flowcontrol "Hardware flow control"; remapctspin "HW Flow control, CTS Pin"; remaprtspin "HW Flow control, RTS Pin"; advanceoptions "Advance options"; rxbuffersize "Rx buffer size (bytes)"; txbuffersize "Tx buffer size (bytes)"; packetmode "Packet mode"; binheader "Binary header (example: '7E 7E')"; binterminator "Binary terminator (example: '03 03')"; porttype_double "Number of data port, type DOUBLE"; porttype_single "Number of data port, type SINGLE"; porttype_int8 "Number of data port, type INT8"; porttype_uint8 "Number of data port, type UINT8"; porttype_int16 "Number of data port, type INT16"; porttype_uint16 "Number of data port, type UINT16"; porttype_int32 "Number of data port, type INT32"; porttype_uint32 "Number of data port, type UINT32"; asciiformat "Ascii format"; rx_asciiterminator "End of packet"; tx_asciiterminator "End of packet"; storagename "Buffer"; varname "Var name"; asciiheader "Ascii header (printf format)"; sampletime "Sample time (sec)"; enablecustomportlabel "Enable custom port labels (Ex. In1, In2, In3)"; cinputportlabel "Custom input port labels (Ex. In1, In2, In3)"; coutputportlabel "Custom output port labels (Ex. Out1, Out2, Out3)"; portpinstr "Port Pin String"; blockid "Block ID"; inputporttype "Input Port Type"; inputportwidth "Input Port Width"; inputportlabel "Input Port Label"; outputporttype "Output Port Type"; outputportwidth "Output Port Width"; outputportlabel "Output port label"; compat "Compatibility (Reserved for future use)"; optionstring "String(s) to be passed to TLC"; lastmodule "Last module selected"
      mask help:
      | UART Module
      |  - Select module corresponding to "UART Setup" block.
      | Transfer
      |  - Blocking: the block wait until data receiving is ready.
      |  - Non-Blocking: if data receiving is ready, the block return non-zero to READY port otherwise return 0.
      | Packet mode:
      |  - Ascii: receiving data is ascii, Ascii format + End of packet.
      |  - Binary: receiving data is binary format, Header + Data + Terminator
      |  - String Buffer: Receiving data stored into Volatile Data Storage variable block.
      | Ascii format:
      |  - %U, %I, %D, %O, %X, %u, %i, %d, %o, %x: Uint32
      |  - %E, %G, %F, %e, %g, %f: Single
      |  - %C, %c: Int8
      mask init:
      | stm32f0_uart_callback('init');
      mask Help: web(fullfile(waijungdocroot,'stm32f0_uart_rx.htm'), '-browser')
      mask StyleString: popup(Setup|Tx|Rx),popup(1|2|3|4),edit,popup(8),popup(No|Odd|Even),popup(0.5|1|1.5|2),popup(Not used|A9|B6),popup(Not used|A10|B7),popup(None|RTS|CTS|RTS/CTS),popup(Not used|A11),popup(Not used|A12),checkbox,popup(16|32|64|128|256|512),popup(16|32|64|128|256|512),popup(Blocking|Non-Blocking),popup(Ascii|Binary|String Buffer),edit,edit,edit,edit,edit,edit,edit,edit,edit,edit,edit,popup(CR (0x0D - "\r")|LF (0x0A - "\n")|CRLF (0x0D 0x0A - "\r\n")),popup(CR (0x0D - "\r")|LF (0x0A - "\n")|CRLF (0x0D 0x0A - "\r\n")|None),popup(<empty>),edit,edit,edit,checkbox,edit,edit,edit,edit,edit,edit,edit,edit,edit,edit,edit,edit,edit,edit,edit,edit
      mask CallbackString: stm32f0_uart_callback('conf');|stm32f0_uart_callback('uartmodule');|||||||stm32f0_uart_callback('flowcontrol');|||stm32f0_uart_callback('advanceoptions');|||stm32f0_uart_callback('conf');|stm32f0_uart_callback('conf');|stm32f0_uart_callback('binheader');|stm32f0_uart_callback('binterminator');|||||||||stm32f0_uart_callback('asciiformat');|||stm32f0_uart_callback('storagename');|||stm32f0_uart_callback('sampletime');|stm32f0_uart_callback('enablecustomportlabel');|stm32f0_uart_callback('conf');|stm32f0_uart_callback('conf');||stm32f0_uart_callback('blockid');||||||||||||
      mask Display: text(0.05, 0.5, 'Module: USART1_Rx\nPacket: Ascii\nTransfer: Non-Blocking\nTs (sec): 0.01','ver','middle','hor','left'); port_label('output', 1,'READY'); port_label('output', 2,'%u');
  wires:
  UART Rx/2 -> Enabled Subsystem/1(In1)
  UART Rx/1 -> Enabled Subsystem/Enable

== system stm32f0_ccp_sensor/CCP Handler/CRO CONNECT Parser/CONNECT Handler ==
  CMD : Inport  OutDataType=fixdt(1, 16)  OutScaling=2^0
  Station Addr LSB : Inport  Port=2  OutDataType=fixdt(1, 16)  OutScaling=2^0
  Station Addr MSB : Inport  Port=3  OutDataType=fixdt(1, 16)  OutScaling=2^0
  CONNECT : simulink/Logic and Bit Operations/Compare To Constant  SystemSampleTime=-1  relop===  const=1  LogicOutDataTypeMode=uint8  ZeroCross=off
  DISCONNECT : simulink/Logic and Bit Operations/Compare To Constant  SystemSampleTime=-1  relop===  const=7  LogicOutDataTypeMode=uint8  ZeroCross=off
  Enabled Subsystem : Subsystem  TreatAsAtomicUnit=on
  Logical Operator : Logic  Operator=OR  AllPortsSameDT=off  OutDataTypeMode=boolean  LogicDataType=fixdt(0, 8)  OutDataTypeStr=boolean
  Connected : Outport  OutDataType=fixdt(1, 16)  OutScaling=2^0
  Station Address : Outport  Port=2  OutDataType=fixdt(1, 16)  OutScaling=2^0
  wires:
  CONNECT/1 -> Logical Operator/1
  DISCONNECT/1 -> Logical Operator/2
  Logical Operator/1 -> Enabled Subsystem/Enable
  CMD/1 -> DISCONNECT/1, CONNECT/1, Enabled Subsystem/1(CMD)
  Enabled Subsystem/1(Connected) -> Connected/1
  Station Addr LSB/1 -> Enabled Subsystem/2(Station address Lsb)
  Station Addr MSB/1 -> Enabled Subsystem/3(Station address Msb)
  Enabled Subsystem/2(Station Addr) -> Station Address/1

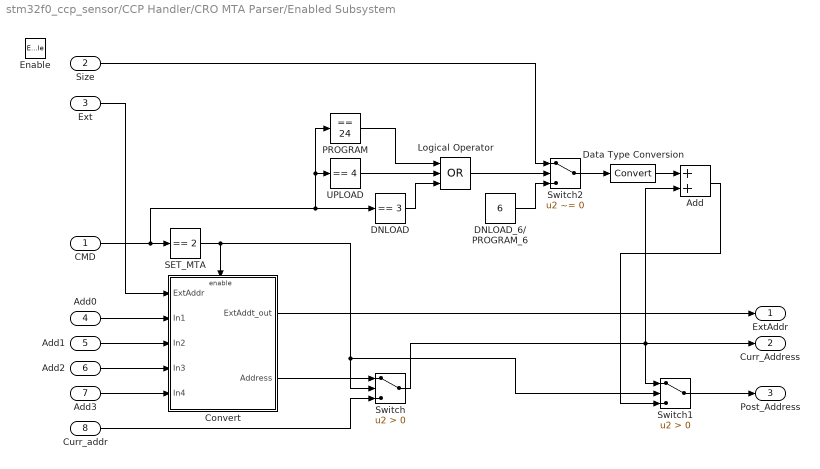
== system stm32f0_ccp_sensor/CCP Handler/CRO MTA Parser/Enabled Subsystem ==
  CMD : Inport  OutDataType=fixdt(1, 16)  OutScaling=2^0
  Size : Inport  Port=2  OutDataType=fixdt(1, 16)  OutScaling=2^0
  Ext : Inport  Port=3  OutDataType=fixdt(1, 16)  OutScaling=2^0
  Add0 : Inport  Port=4  OutDataType=fixdt(1, 16)  OutScaling=2^0
  Add1 : Inport  Port=5  OutDataType=fixdt(1, 16)  OutScaling=2^0
  Add2 : Inport  Port=6  OutDataType=fixdt(1, 16)  OutScaling=2^0
  Add3 : Inport  Port=7  OutDataType=fixdt(1, 16)  OutScaling=2^0
  Curr_addr : Inport  Port=8  OutDataType=fixdt(1, 16)  OutScaling=2^0
  Enable : EnablePort
  Add : Sum  OutDataType=fixdt(1, 16)  OutScaling=2^-10
  Convert : Subsystem  TreatAsAtomicUnit=on
  DNLOAD : simulink/Logic and Bit Operations/Compare To Constant  SystemSampleTime=-1  relop===  const=3  LogicOutDataTypeMode=uint8  ZeroCross=off
  DNLOAD_6/ PROGRAM_6 : Constant  Value=6  OutDataTypeMode=uint8  OutDataType=fixdt(1, 16)  OutScaling=2^0  OutDataTypeStr=uint8
  Data Type Conversion : DataTypeConversion  OutDataType=fixdt(1, 16)  OutScaling=2^0
  Logical Operator : Logic  Operator=OR  Inputs=3  AllPortsSameDT=off  OutDataTypeMode=boolean  LogicDataType=fixdt(0, 8)  OutDataTypeStr=boolean
  PROGRAM : simulink/Logic and Bit Operations/Compare To Constant  SystemSampleTime=-1  relop===  const=24  LogicOutDataTypeMode=uint8  ZeroCross=off
  SET_MTA : simulink/Logic and Bit Operations/Compare To Constant  SystemSampleTime=-1  relop===  const=2  LogicOutDataTypeMode=uint8  ZeroCross=off
  Switch : Switch  Criteria=u2 > Threshold  OutDataType=fixdt(1, 16)  OutScaling=2^0
  Switch1 : Switch  Criteria=u2 > Threshold  OutDataType=fixdt(1, 16)  OutScaling=2^0
  Switch2 : Switch  Criteria=u2 ~= 0  OutDataType=fixdt(1, 16)  OutScaling=2^0
  UPLOAD : simulink/Logic and Bit Operations/Compare To Constant  SystemSampleTime=-1  relop===  const=4  LogicOutDataTypeMode=uint8  ZeroCross=off
  ExtAddr : Outport  OutDataType=fixdt(1, 16)  OutScaling=2^0  InitialOutput=0
  Curr_Address : Outport  Port=2  OutDataType=fixdt(1, 16)  OutScaling=2^0  InitialOutput=0
  Post_Address : Outport  Port=3  OutDataType=fixdt(1, 16)  OutScaling=2^0  InitialOutput=0
  wires:
  CMD/1 -> SET_MTA/1, DNLOAD/1, UPLOAD/1, PROGRAM/1
  Add0/1 -> Convert/2(In1)
  Add1/1 -> Convert/3(In2)
  Add2/1 -> Convert/4(In3)
  Add3/1 -> Convert/5(In4)
  SET_MTA/1 -> Convert/Enable, Switch/2, Switch1/2
  Convert/2(Address) -> Switch/1
  Switch/1 -> Curr_Address/1, Switch1/1, Add/2
  Logical Operator/1 -> Switch2/2
  Ext/1 -> Convert/1(ExtAddr)
  DNLOAD_6/ PROGRAM_6/1 -> Switch2/3
  Switch2/1 -> Data Type Conversion/1
  Add/1 -> Switch1/3
  DNLOAD/1 -> Logical Operator/3
  UPLOAD/1 -> Logical Operator/2
  PROGRAM/1 -> Logical Operator/1
  Data Type Conversion/1 -> Add/1
  Curr_addr/1 -> Switch/3
  Switch1/1 -> Post_Address/1
  Convert/1(ExtAddt_out) -> ExtAddr/1
  Size/1 -> Switch2/1

== system stm32f0_ccp_sensor/CCP Handler/CRO MTA Parser/Hold Valid Addr ==
  In1 : Inport
  In2 : Inport  Port=2
  In3 : Inport  Port=3
  Enable : EnablePort
  ExtAddr : Outport  OutDataType=fixdt(1, 16)  OutScaling=2^0  InitialOutput=0
  MTA : Outport  Port=2  OutDataType=fixdt(1, 16)  OutScaling=2^0  InitialOutput=0
  Post_MTA : Outport  Port=3  OutDataType=fixdt(1, 16)  OutScaling=2^0  InitialOutput=0
  wires:
  In3/1 -> Post_MTA/1
  In1/1 -> ExtAddr/1
  In2/1 -> MTA/1

== system stm32f0_ccp_sensor/CCP Handler/CRO MTA Parser/Validate Base Address ==
  ExtAddr : Inport
  PostInc : Inport  Port=2
  Compare To Constant : simulink/Logic and Bit Operations/Compare To Constant  SystemSampleTime=-1  relop=<=  const=4  LogicOutDataTypeMode=uint8  ZeroCross=off
  Demux : Demux  Outputs=2
  INVALID_EXTADDR : Constant  Value=0  OutDataTypeMode=uint8  OutDataType=fixdt(1, 16)  OutScaling=2^0  OutDataTypeStr=uint8
  Interval Test Dynamic : simulink/Logic and Bit Operations/Interval Test Dynamic  SystemSampleTime=-1  IntervalClosedRight=on  IntervalClosedLeft=on  LogicOutDataTypeMode=uint8
  Limit EXT_0 (ID) : Constant  Value=[16 0]  OutDataTypeMode=uint32  OutDataType=fixdt(1, 16)  OutScaling=2^0  OutDataTypeStr=uint32
  Limit EXT_1 (RO) : Constant  Value=[255 0]  OutDataTypeMode=uint32  OutDataType=fixdt(1, 16)  OutScaling=2^0  OutDataTypeStr=uint32
  Limit EXT_2 (RW) : Constant  Value=[255 0]  OutDataTypeMode=uint32  OutDataType=fixdt(1, 16)  OutScaling=2^0  OutDataTypeStr=uint32
  Limit EXT_3 (FLASH) : Constant  Value=[52*1024 0]  OutDataTypeMode=uint32  OutDataType=fixdt(1, 16)  OutScaling=2^0  OutDataTypeStr=uint32
  Limit EXT_4 (EEPROM) : Constant  Value=[255 0]  OutDataTypeMode=uint32  OutDataType=fixdt(1, 16)  OutScaling=2^0  OutDataTypeStr=uint32
  Multiport Switch : MultiPortSwitch  Inputs=5  zeroidx=on  OutDataType=fixdt(1, 16)  OutScaling=2^0
  Saturation : Saturate  UpperLimit=4  LowerLimit=0  OutDataType=fixdt(1, 16)  OutScaling=2^0
  Switch : Switch  Criteria=u2 ~= 0  OutDataType=fixdt(1, 16)  OutScaling=2^0
  ValidAddr : Outport  OutDataType=fixdt(1, 16)  OutScaling=2^0
  wires:
  ExtAddr/1 -> Compare To Constant/1, Saturation/1
  Compare To Constant/1 -> Switch/2
  INVALID_EXTADDR/1 -> Switch/3
  Limit EXT_0 (ID)/1 -> Multiport Switch/2
  Limit EXT_1 (RO)/1 -> Multiport Switch/3
  Limit EXT_2 (RW)/1 -> Multiport Switch/4
  Limit EXT_3 (FLASH)/1 -> Multiport Switch/5
  Limit EXT_4 (EEPROM)/1 -> Multiport Switch/6
  PostInc/1 -> Interval Test Dynamic/2
  Multiport Switch/1 -> Demux/1
  Interval Test Dynamic/1 -> Switch/1
  Switch/1 -> ValidAddr/1
  Demux/1 -> Interval Test Dynamic/1
  Demux/2 -> Interval Test Dynamic/3
  Saturation/1 -> Multiport Switch/1

== system stm32f0_ccp_sensor/CCP Handler/CRO UNLOCK Parser/Enabled Subsystem ==
  CMD : Inport  OutDataType=fixdt(1, 16)  OutScaling=2^0
  Data(6) : Inport  Port=2  OutDataType=fixdt(1, 16)  OutScaling=2^0
  Last status : Inport  Port=3  OutDataType=fixdt(1, 16)  OutScaling=2^0
  Enable : EnablePort
  Enabled Subsystem : Subsystem  TreatAsAtomicUnit=on
  Switch : Switch  Criteria=u2 > Threshold  OutDataType=fixdt(1, 16)  OutScaling=2^0
  UNLOCK : simulink/Logic and Bit Operations/Compare To Constant  SystemSampleTime=-1  relop===  const=19  LogicOutDataTypeMode=uint8  ZeroCross=off
  Out1 : Outport  OutDataType=fixdt(1, 16)  OutScaling=2^0
  wires:
  CMD/1 -> UNLOCK/1
  UNLOCK/1 -> Switch/2, Enabled Subsystem/Enable
  Last status/1 -> Switch/3, Enabled Subsystem/2(Last state)
  Switch/1 -> Out1/1
  Data(6)/1 -> Enabled Subsystem/1(In1)
  Enabled Subsystem/1(Out1) -> Switch/1

== system stm32f0_ccp_sensor/CCP Handler/Command Processing/BUILD_CHKSUM ==
  CMD : Inport
  CTR : Inport  Port=2
  Data(6) : Inport  Port=3
  MTA : Inport  Port=4
  Unlock status : Inport  Port=5
  BUILD_CHKSUM : simulink/Logic and Bit Operations/Compare To Constant  SystemSampleTime=-1  relop===  const=14  LogicOutDataTypeMode=uint8  ZeroCross=off
  BUILD_CHKSUM Handler : Subsystem  TreatAsAtomicUnit=on
  Valid : Outport
  Data (8) : Outport  Port=2
  wires:
  BUILD_CHKSUM/1 -> BUILD_CHKSUM Handler/Enable, Valid/1
  CMD/1 -> BUILD_CHKSUM/1
  CTR/1 -> BUILD_CHKSUM Handler/1(CTR)
  BUILD_CHKSUM Handler/1(Out1) -> Data (8)/1
  Data(6)/1 -> BUILD_CHKSUM Handler/2(Data(6))
  MTA/1 -> BUILD_CHKSUM Handler/3(MTA)
  Unlock status/1 -> BUILD_CHKSUM Handler/4(Unlock status)

== system stm32f0_ccp_sensor/CCP Handler/Command Processing/CLEAR_MEMORY ==
  CMD : Inport
  CTR : Inport  Port=2
  Data(6) : Inport  Port=3
  MTA : Inport  Port=4
  Unlock status : Inport  Port=5
  CLEAR_MEMORY : simulink/Logic and Bit Operations/Compare To Constant  SystemSampleTime=-1  relop===  const=16  LogicOutDataTypeMode=uint8  ZeroCross=off
  CLEAR_MEMORY Handler : Subsystem  TreatAsAtomicUnit=on
  Valid : Outport
  Data (8) : Outport  Port=2
  wires:
  Unlock status/1 -> CLEAR_MEMORY Handler/4(Unlock status)
  Data(6)/1 -> CLEAR_MEMORY Handler/2(Data(6))
  CLEAR_MEMORY Handler/1(Out1) -> Data (8)/1
  CTR/1 -> CLEAR_MEMORY Handler/1(CTR)
  CMD/1 -> CLEAR_MEMORY/1
  CLEAR_MEMORY/1 -> Valid/1, CLEAR_MEMORY Handler/Enable
  MTA/1 -> CLEAR_MEMORY Handler/3(MTA)

== system stm32f0_ccp_sensor/CCP Handler/Command Processing/CONNECT ==
  CMD : Inport
  CTR : Inport  Port=2
  CONNECT : simulink/Logic and Bit Operations/Compare To Constant  SystemSampleTime=-1  relop===  const=1  LogicOutDataTypeMode=uint8  ZeroCross=off
  CONNECT Handler : Subsystem  TreatAsAtomicUnit=on
  Valid : Outport
  Data (8) : Outport  Port=2
  wires:
  CONNECT/1 -> CONNECT Handler/Enable, Valid/1
  CMD/1 -> CONNECT/1
  CTR/1 -> CONNECT Handler/1(CTR)
  CONNECT Handler/1(Out1) -> Data (8)/1

== system stm32f0_ccp_sensor/CCP Handler/Command Processing/DISCONNECT ==
  CMD : Inport
  CTR : Inport  Port=2
  Unlock status : Inport  Port=3
  DISCONNECT : simulink/Logic and Bit Operations/Compare To Constant  SystemSampleTime=-1  relop===  const=7  LogicOutDataTypeMode=uint8  ZeroCross=off
  DISCONNECT Handler : Subsystem  TreatAsAtomicUnit=on
  Logical Operator : Logic  AllPortsSameDT=off  OutDataTypeMode=boolean  LogicDataType=fixdt(0, 8)  OutDataTypeStr=boolean
  Valid : Outport
  Data (8) : Outport  Port=2
  Reset : Outport  Port=3
  wires:
  DISCONNECT Handler/1(Out1) -> Data (8)/1
  CTR/1 -> DISCONNECT Handler/1(CTR)
  CMD/1 -> DISCONNECT/1
  DISCONNECT/1 -> DISCONNECT Handler/Enable, Valid/1, Logical Operator/1
  Unlock status/1 -> DISCONNECT Handler/2(Unlock status)
  DISCONNECT Handler/2(Reset) -> Logical Operator/2
  Logical Operator/1 -> Reset/1

== system stm32f0_ccp_sensor/CCP Handler/Command Processing/DNLOAD/DNLOAD_6 ==
  CMD : Inport
  CTR : Inport  Port=2
  MTA : Inport  Port=3
  Data(6) : Inport  Port=4
  DOWNLOAD : simulink/Logic and Bit Operations/Compare To Constant  SystemSampleTime=-1  relop===  const=3  LogicOutDataTypeMode=uint8  ZeroCross=off
  DOWNLOAD/DOWNLOAD_6 Handler : Subsystem  TreatAsAtomicUnit=on
  DOWNLOAD_6 : simulink/Logic and Bit Operations/Compare To Constant  SystemSampleTime=-1  relop===  const=35  LogicOutDataTypeMode=uint8  ZeroCross=off
  Data Type Conversion : DataTypeConversion  OutDataTypeMode=uint8  OutDataType=fixdt(1, 16)  OutScaling=2^0  OutDataTypeStr=uint8
  Logical Operator : Logic  Operator=OR  AllPortsSameDT=off  OutDataTypeMode=boolean  LogicDataType=fixdt(0, 8)  OutDataTypeStr=boolean
  Valid : Outport
  Data (8) : Outport  Port=2
  wires:
  DOWNLOAD/DOWNLOAD_6 Handler/1(Out1) -> Data (8)/1
  CTR/1 -> DOWNLOAD/DOWNLOAD_6 Handler/2(CTR)
  CMD/1 -> DOWNLOAD/1, DOWNLOAD_6/1, DOWNLOAD/DOWNLOAD_6 Handler/1(CMD)
  Data(6)/1 -> DOWNLOAD/DOWNLOAD_6 Handler/4(Data(6))
  MTA/1 -> DOWNLOAD/DOWNLOAD_6 Handler/3(MTA)
  DOWNLOAD/1 -> Logical Operator/1
  DOWNLOAD_6/1 -> Logical Operator/2
  Logical Operator/1 -> DOWNLOAD/DOWNLOAD_6 Handler/Enable, Data Type Conversion/1
  Data Type Conversion/1 -> Valid/1

== system stm32f0_ccp_sensor/CCP Handler/Command Processing/EXCHANGE_ID ==
  CMD : Inport
  CTR : Inport  Port=2
  EXCHANGE_ID : simulink/Logic and Bit Operations/Compare To Constant  SystemSampleTime=-1  relop===  const=23  LogicOutDataTypeMode=uint8  ZeroCross=off
  EXCHANGE_ID Handler : Subsystem  TreatAsAtomicUnit=on
  Valid : Outport
  Data (8) : Outport  Port=2
  wires:
  EXCHANGE_ID Handler/1(Out1) -> Data (8)/1
  CTR/1 -> EXCHANGE_ID Handler/1(CTR)
  CMD/1 -> EXCHANGE_ID/1
  EXCHANGE_ID/1 -> Valid/1, EXCHANGE_ID Handler/Enable

== system stm32f0_ccp_sensor/CCP Handler/Command Processing/GET_SEED ==
  CMD : Inport
  CTR : Inport  Port=2
  Data(6) : Inport  Port=3
  Unlock status : Inport  Port=4
  GET_SEED : simulink/Logic and Bit Operations/Compare To Constant  SystemSampleTime=-1  relop===  const=18  LogicOutDataTypeMode=uint8  ZeroCross=off
  GET_SEED Handler : Subsystem  TreatAsAtomicUnit=on
  Valid : Outport
  Data (8) : Outport  Port=2
  wires:
  GET_SEED/1 -> GET_SEED Handler/Enable, Valid/1
  CMD/1 -> GET_SEED/1
  CTR/1 -> GET_SEED Handler/1(CTR)
  GET_SEED Handler/1(Out1) -> Data (8)/1
  Data(6)/1 -> GET_SEED Handler/2(Data(6))
  Unlock status/1 -> GET_SEED Handler/3(Unlock status)

== system stm32f0_ccp_sensor/CCP Handler/Command Processing/PROGRAM/ PROGRAM_6 ==
  CMD : Inport
  CTR : Inport  Port=2
  Data(6) : Inport  Port=3
  MTA : Inport  Port=4
  Unlock status : Inport  Port=5
  Data Type Conversion : DataTypeConversion  OutDataTypeMode=uint8  OutDataType=fixdt(1, 16)  OutScaling=2^0  OutDataTypeStr=uint8
  Logical Operator : Logic  Operator=OR  AllPortsSameDT=off  OutDataTypeMode=boolean  LogicDataType=fixdt(0, 8)  OutDataTypeStr=boolean
  PROGRAM : simulink/Logic and Bit Operations/Compare To Constant  SystemSampleTime=-1  relop===  const=24  LogicOutDataTypeMode=uint8  ZeroCross=off
  PROGRAM/PROGRAM_6 Handler : Subsystem  TreatAsAtomicUnit=on
  PROGRAM_6 : simulink/Logic and Bit Operations/Compare To Constant  SystemSampleTime=-1  relop===  const=34  LogicOutDataTypeMode=uint8  ZeroCross=off
  Valid : Outport
  Data (8) : Outport  Port=2
  wires:
  CMD/1 -> PROGRAM/1, PROGRAM_6/1, PROGRAM/PROGRAM_6 Handler/1(CMD)
  CTR/1 -> PROGRAM/PROGRAM_6 Handler/2(CTR)
  PROGRAM/PROGRAM_6 Handler/1(Out1) -> Data (8)/1
  Data(6)/1 -> PROGRAM/PROGRAM_6 Handler/3(Data(6))
  Unlock status/1 -> PROGRAM/PROGRAM_6 Handler/5(Unlock status)
  PROGRAM_6/1 -> Logical Operator/2
  PROGRAM/1 -> Logical Operator/1
  Logical Operator/1 -> PROGRAM/PROGRAM_6 Handler/Enable, Data Type Conversion/1
  MTA/1 -> PROGRAM/PROGRAM_6 Handler/4(MTA)
  Data Type Conversion/1 -> Valid/1

== system stm32f0_ccp_sensor/CCP Handler/Command Processing/SET_MTA ==
  CMD : Inport
  CTR : Inport  Port=2
  MTA : Inport  Port=3
  SET_MTA : simulink/Logic and Bit Operations/Compare To Constant  SystemSampleTime=-1  relop===  const=2  LogicOutDataTypeMode=uint8  ZeroCross=off
  SET_MTA Handler : Subsystem  TreatAsAtomicUnit=on
  Valid : Outport
  Data (8) : Outport  Port=2
  wires:
  SET_MTA/1 -> SET_MTA Handler/Enable, Valid/1
  CMD/1 -> SET_MTA/1
  CTR/1 -> SET_MTA Handler/1(CTR)
  SET_MTA Handler/1(Out1) -> Data (8)/1
  MTA/1 -> SET_MTA Handler/2(MTA)

== system stm32f0_ccp_sensor/CCP Handler/Command Processing/SHORT_UP ==
  CMD : Inport
  CTR : Inport  Port=2
  Data(6) : Inport  Port=3
  SHORT_UP : simulink/Logic and Bit Operations/Compare To Constant  SystemSampleTime=-1  relop===  const=15  LogicOutDataTypeMode=uint8  ZeroCross=off
  SHORT_UP Handler : Subsystem  TreatAsAtomicUnit=on
  Valid : Outport
  Data (8) : Outport  Port=2
  wires:
  CTR/1 -> SHORT_UP Handler/1(CTR)
  CMD/1 -> SHORT_UP/1
  SHORT_UP/1 -> Valid/1, SHORT_UP Handler/Enable
  Data(6)/1 -> SHORT_UP Handler/2(Data(6))
  SHORT_UP Handler/1(Out1) -> Data (8)/1

== system stm32f0_ccp_sensor/CCP Handler/Command Processing/UNLOCK ==
  CMD : Inport
  CTR : Inport  Port=2
  Unlock status : Inport  Port=3
  UNLOCK : simulink/Logic and Bit Operations/Compare To Constant  SystemSampleTime=-1  relop===  const=19  LogicOutDataTypeMode=uint8  ZeroCross=off
  UNLOCK Handler : Subsystem  TreatAsAtomicUnit=on
  Valid : Outport
  Data (8) : Outport  Port=2
  wires:
  UNLOCK Handler/1(Out1) -> Data (8)/1
  CTR/1 -> UNLOCK Handler/1(CTR)
  CMD/1 -> UNLOCK/1
  UNLOCK/1 -> Valid/1, UNLOCK Handler/Enable
  Unlock status/1 -> UNLOCK Handler/2(Unlock status)

== system stm32f0_ccp_sensor/CCP Handler/Command Processing/UPLOAD ==
  CMD : Inport
  CTR : Inport  Port=2
  MTA : Inport  Port=3
  Data(6) : Inport  Port=4
  DOWNLOAD : simulink/Logic and Bit Operations/Compare To Constant  SystemSampleTime=-1  relop===  const=4  LogicOutDataTypeMode=uint8  ZeroCross=off
  UPLOAD : Subsystem  TreatAsAtomicUnit=on
  Valid : Outport
  Data (8) : Outport  Port=2
  wires:
  DOWNLOAD/1 -> UPLOAD/Enable, Valid/1
  MTA/1 -> UPLOAD/2(MTA)
  Data(6)/1 -> UPLOAD/3(Data(6))
  CMD/1 -> DOWNLOAD/1
  CTR/1 -> UPLOAD/1(CTR)
  UPLOAD/1(Out1) -> Data (8)/1
